simulink model "Copy_of_rotary_system_23a"  (R2023a)
settings: Solver=ode1  StartTime=0.0  StopTime=0.15  FixedStep=1e-7  MaxStep=1e-5  RelTol=1e-6
InitFcn:
  | %% Parameters
  | 
  | param = struct();
  | 
  | % Volume of chambers
  | param.V1_0 = 1e-3;
  | param.V2_0 = 20e-6;
  | 
  | % Pressure rails
  | param.P_H = 20e6;
  | param.P_M = 10e6;
  | 
  | % Valve things
  | param.max_Avt = 0.5*0.25*pi*(20e-3)^2;
  | param.Cd = 0.6;
  | 
  | % Fluid properties
  | param.beta = 1.8e9;
  | param.rho = 870;
  | 
  | % Electric motor stuff
  | param.Kt = 70.5e-3;
  | param.Ke = 70.5e-3;
  | param.J_elec = 140e-7;
  | 
  | % Pump things
  | param.J_hyd = 3000e-7;
  | param.hyd_D = 1.6e-6;    % In cc/rev
  | 
  | % Simulation time
  | T = 1;
settings Model: Creator=user  LastModifiedBy=ibrah408

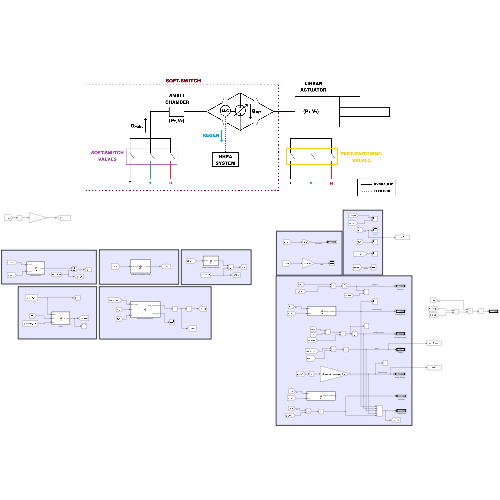
[thumbnail: Simulink's stored preview of the top-level diagram]
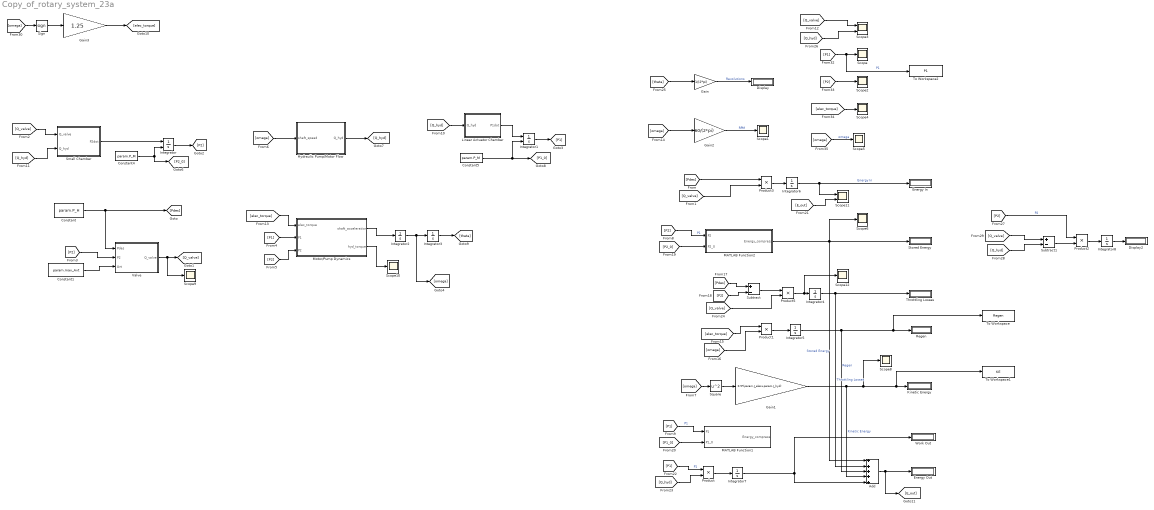
== system Copy_of_rotary_system_23a ==
  Add : Sum  Inputs=+++++
  Constant : Constant  Value=param.P_H
  Constant1 : Constant  Value=param.max_Avt
  Constant4 : Constant  Value=param.P_M
  Constant5 : Constant  Value=param.P_M
  Display : Display
  Display2 : Display
  Energy In : Display
  Energy Out : Display
  Gain : Gain  Gain=1/(2*pi)
  Gain1 : Gain  Gain=0.5*(param.J_elec+param.J_hyd)
  Gain2 : Gain  Gain=60/(2*pi)
  Gain3 : Gain  Gain=1.25
  Hydraulic Pump/Motor Flow : MATLAB Function  TreatAsAtomicUnit=on
  Integrator : Integrator  InitialConditionSource=external  InitialCondition=param.P_M
  Integrator1 : Integrator  InitialConditionSource=external  InitialCondition=param.P_M
  Integrator{2..8} (7 alike) : Integrator
  Kinetic Energy : Display
  Linear Actuator Chamber : MATLAB Function  TreatAsAtomicUnit=on
  MATLAB Function1 : MATLAB Function  TreatAsAtomicUnit=on
  MATLAB Function2 : MATLAB Function  TreatAsAtomicUnit=on
  Motor/Pump Dynamics : MATLAB Function  TreatAsAtomicUnit=on
  Product{,1..3,5} (5 alike) : Product
  Regen : Display
  Scope{,1..2,4..6,8..10,12} (10 alike) : Scope
  Scope11 : Scope  NumInputPorts=2
  Scope3 : Scope  NumInputPorts=2
  Sign : Signum
  Small Chamber : MATLAB Function  TreatAsAtomicUnit=on
  Square : Math  Operator=square
  Stored Energy : Display
  Subtract : Sum  Inputs=+-
  Subtract1 : Sum  Inputs=+-
  Throttling Losses : Display
  To Workspace : ToWorkspace  VariableName=Regen  SaveFormat=Timeseries  SampleTime=-1
  To Workspace1 : ToWorkspace  VariableName=KE  SaveFormat=Timeseries  SampleTime=-1
  To Workspace2 : ToWorkspace  VariableName=P1  SaveFormat=Timeseries  SampleTime=-1
  Valve : MATLAB Function  TreatAsAtomicUnit=on
  Work Out : Display
  wires:
  Small Chamber/1(P2dot) -> Integrator/1
  Linear Actuator Chamber/1(P1dot) -> Integrator1/1
  Integrator/1 -> [P2]
  Integrator1/1 -> [P1]
  Motor/Pump Dynamics/1(shaft_acceleration) -> Integrator2/1
  Integrator2/1 -> Integrator3/1, [omega]
  Hydraulic Pump/Motor Flow/1(Q_hyd) -> [Q_hyd]
  Gain2/1 -> Scope1/1  "RPM"
  Constant1/1 -> Valve/3(Avt)
  Valve/1(Q_valve) -> Scope9/1, [Q_valve]
  [Q_valve] -> Small Chamber/1(Q_valve)
  [P2] -> Valve/2(P2)
  [omega] -> Hydraulic Pump/Motor Flow/1(shaft_speed)
  [Q_hyd] -> Small Chamber/2(Q_hyd)
  [Q_hyd] -> Linear Actuator Chamber/1(Q_hyd)
  [elec_torque] -> Motor/Pump Dynamics/1(elec_torque)
  [omega] -> Gain2/1
  Integrator6/1 -> Scope11/1, Energy In/1  "Energy In"
  MATLAB Function2/1(Energy_compress) -> Add/1, Scope6/1, Stored Energy/1  "Stored Energy"
  Gain1/1 -> Scope8/1, To Workspace1/1, Kinetic Energy/1, Add/4  "Kinetic Energy"
  Subtract/1 -> Product5/1
  [Q_valve] -> Product3/2
  Integrator5/1 -> Add/3, To Workspace/1, Regen/1  "Regen"
  [omega] -> Product1/2
  Product1/1 -> Integrator5/1
  [P2] -> Subtract/2
  Product3/1 -> Integrator6/1
  [Q_valve] -> Product5/2
  [Pdes] -> Subtract/1
  [elec_torque] -> Product1/1
  [Pdes] -> Product3/1
  Product5/1 -> Scope12/1, Integrator4/1
  Integrator4/1 -> Throttling Losses/1, Add/2  "Throttling Losses"
  Add/1 -> [E_out], Energy Out/1
  Gain/1 -> Display/1  "Revolutions"
  Integrator3/1 -> [theta]
  [theta] -> Gain/1
  [P2] -> Scope2/1
  [elec_torque] -> Scope4/1
  [omega] -> Scope5/1  "omega"
  Constant/1 -> Valve/1(Pdes), [Pdes]
  [Q_valve] -> Scope3/1
  [Q_hyd] -> Scope3/2
  [omega] -> Square/1
  Square/1 -> Gain1/1
  [P1] -> Motor/Pump Dynamics/2(P1)
  [P2] -> Motor/Pump Dynamics/3(P2)
  Motor/Pump Dynamics/2(hyd_torque) -> Scope10/1
  [P1] -> To Workspace2/1, Scope/1  "P1"
  [P1] -> MATLAB Function1/1(P1)  "P1"
  Constant4/1 -> Integrator/2, [P2_0]
  Constant5/1 -> [P1_0], Integrator1/2
  [P1_0] -> MATLAB Function1/2(P1_0)
  [P2_0] -> MATLAB Function2/2(P2_0)
  [P2] -> MATLAB Function2/1(P2)  "P1"
  [E_out] -> Scope11/2
  [P1] -> Product/1  "P1"
  [Q_hyd] -> Product/2
  Product/1 -> Integrator7/1
  Integrator7/1 -> Add/5, Work Out/1
  [Q_valve] -> Subtract1/1
  [Q_hyd] -> Subtract1/2
  Integrator8/1 -> Display2/1
  Subtract1/1 -> Product2/2
  [P2] -> Product2/1  "P2"
  Product2/1 -> Integrator8/1
  [omega] -> Sign/1
  Gain3/1 -> [elec_torque]
  Sign/1 -> Gain3/1

== matlab function Copy_of_rotary_system_23a/Small Chamber ==
  data: P2dot output; param parameter; Q_valve input; Q_hyd input
function P2dot = fcn(param, Q_valve, Q_hyd)

P2dot = (param.beta/param.V2_0)*(Q_valve - Q_hyd);

== matlab function Copy_of_rotary_system_23a/Valve ==
  data: Q_valve output; Pdes input; P2 input; Avt input; param parameter
function Q_valve = fcn(Pdes, P2, Avt, param)

Q_valve = param.Cd*Avt*sqrt((2/param.rho)*abs(Pdes-P2))*sign(Pdes-P2);

== matlab function Copy_of_rotary_system_23a/Hydraulic Pump//Motor Flow ==
  data: Q_hyd output; param parameter; shaft_speed input
function Q_hyd  = fcn(param, shaft_speed)

Q_hyd = (param.hyd_D/(2*pi))*shaft_speed;

== matlab function Copy_of_rotary_system_23a/MATLAB Function2 ==
  data: P2 input; P2_0 input; Energy_compress output; param parameter
function Energy_compress  = fcn(P2, P2_0, param)

%% Normal
Wv = param.beta*(exp(P2/param.beta)-(1+P2/param.beta));
W0 = param.beta*(exp(P2_0/param.beta)-(1+P2_0/param.beta));

Energy_compress = param.V2_0*(Wv-W0);

%% Hydraulic Effort
% phi_v = param.beta*(exp(P2/param.beta)-1);
% phi_0 = param.beta*(exp(P2_0/param.beta)-1);

% Energy_compress = param.V2_0*(phi_v-phi_0);

== matlab function Copy_of_rotary_system_23a/Linear Actuator Chamber ==
  data: P1dot output; param parameter; Q_hyd input
function P1dot = fcn(param, Q_hyd)

P1dot = (param.beta/param.V1_0)*(Q_hyd);

== matlab function Copy_of_rotary_system_23a/Motor//Pump Dynamics ==
  data: shaft_acceleration output; param parameter; elec_torque input; P1 input; P2 input; hyd_torque output
function [shaft_acceleration, hyd_torque] = fcn(param, elec_torque, P1, P2)

hyd_torque = (param.hyd_D/(2*pi))*(P2 - P1);

shaft_acceleration = (1/(param.J_hyd+param.J_elec))*(hyd_torque - elec_torque);

== matlab function Copy_of_rotary_system_23a/MATLAB Function1 ==
  data: P1 input; P1_0 input; Energy_compress output; param parameter
function Energy_compress = fcn(P1, P1_0, param)

Wv = param.beta*(exp(P1/param.beta)-(1+P1/param.beta));
W0 = param.beta*(exp(P1_0/param.beta)-(1+P1_0/param.beta));

Energy_compress = param.V1_0*(Wv-W0);
